simulink model "general_charger_2_precharge"  (R2013a)
settings: Solver=ode23  StartTime=0  StopTime=1.5  RelTol=1e-3
PreLoadFcn:
  | Ts =5e-6;
values from neighbouring files (symbols this model uses):
  ac_volt = 169    [charger_init.m]    (also in charger_init_simpl.m)
  acdc_on_time = 0.2    [charger_init.m]    (also in charger_init_simpl.m = 0)
  Cdc = 2e-3    (= 0.002)    [charger_init.m]    (also in charger_init_simpl.m)
  dcAd = dcinvexp*(eye(dcnstates) + (Ts/2)*dcAc)    [charger_init.m]    (also in charger_init_simpl.m)
  dcBd = dcinvexp*dcBc    [charger_init.m]    (also in charger_init_simpl.m)
  dcCd = dcCc*dcinvexp*Ts    [charger_init.m]    (also in charger_init_simpl.m)
  dcDd = dcCc*dcinvexp*dcBc*(Ts/2) + dcDc    [charger_init.m]    (also in charger_init_simpl.m)
  ESRCd = 70e-3    (= 0.07)    [charger_init.m]    (also in charger_init_simpl.m)
  ESRLdcdc = 0.1    [charger_init.m]    (also in charger_init_simpl.m)
  ESRLin = 0.2    [charger_init.m]    (also in charger_init_simpl.m = 0.1)
  Ldcdc = 1.3e-3    (= 0.0013)    [charger_init.m]    (also in charger_init_simpl.m = 0.0014)
  Lin = 1.5e-3    (= 0.0015)    [charger_init.m]    (also in charger_init_simpl.m = 0.001)
  P = 1.92e3    (= 1920)    [charger_init.m]    (also in charger_init_simpl.m)
  pre_charge_off = 0.2    [charger_init.m]
  pre_charge_r = 10    [charger_init.m]    (also in charger_init_simpl.m = 6)
  pre_charge_ramp = (dc_volt - Vdcmin)/(acdc_ramp_end_time - acdc_on_time)    (= 336.666666667)    [charger_init.m]    (also in charger_init_simpl.m = (dc_volt - Vdcmin)/(acdc_ramp_end_time - acdc_on_time))
  Q = 0    [charger_init.m]    (also in charger_init_simpl.m)
  Rbatt = 0.20    (= 0.2)    [charger_init.m]    (also in charger_init_simpl.m = 0.1)
  switch_Ts = 5e-5    (= 5e-05)    [charger_init.m]    (also in charger_init_simpl.m)
  sys_Ts = 5e-6    (= 5e-06)    [charger_init.m]    (also in charger_init_simpl.m)
  Vdcmin = ac_volt + 10    (= 179)    [charger_init.m]    (also in charger_init_simpl.m)
  voc = 105    [charger_init.m]    (also in charger_init_simpl.m)
undefined symbols (not defined in the file or in its folder): cpi
undefined symbols (not defined in the file): active_power_on, Ad, Bd, Cd, dc_volt, dcdc_cc_ref, dcdc_cv_ref, dcdc_iki, dcdc_ikp, dcdc_on, dcdc_vki, dcdc_vkp, Dd, dq_id_ki, dq_id_kp, dq_iq_ki, dq_iq_kp, dq_vdc_ki, dq_vdc_kp, dqQ_ki, dqQ_kp, P_ki, P_kp, pi_iac_ki, pi_iac_kp, pi_vdc_ki, pi_vdc_kp, piQ_ki, piQ_kp, pr_iac_kp, pr_pr_ki, pr_pr_kp, pr_vdc_ki, pr_vdc_kp, reactive_power_on
libraries: simulink_extras x165, powerlib x64, simulink x35, powerlib_meascontrol x11
(part 1 of 7)
settings Model: Creator=Administrator  LastModifiedBy=jfmorris
settings DataIOCC: SaveFinalState=on  SignalLoggingSaveFormat=ModelDataLogs
settings OptimizationCC: ExpressionDepthLimit=2147483647
settings DebuggingCC: FcnCallInpInsideContextMsg=UseLocalSettings  UnconnectedLineMsg=none
settings GRTTargetCC: CombineOutputUpdateFcns=off  GRTInterface=on

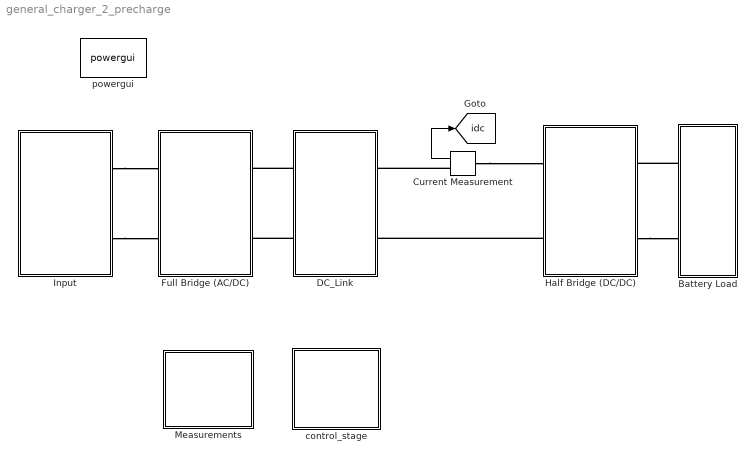
== system general_charger_2_precharge ==
  Battery Load : Subsystem
  Current Measurement : powerlib/Measurements/Current Measurement  PhasorSimulation=off  OutputType=Complex  PSBequivalent=0
  DC_Link : Subsystem
  Full Bridge (AC/DC) : Subsystem  mask{rsnub=50e3, csnub=0.33e-6, ron=1e-3, c_bridge=1e-6}
      mask prompts: rsnub "Snubber Resistance, ohms"; csnub "Snubber Capacitance, F"; ron "On Resistance, ohms"; c_bridge "Bridge Capacitance, F"
  Half Bridge (DC/DC) : Subsystem  mask{rsnub=50e3, csnub=1e-6, ron=1e-3, c_bridge=1e-6}
      mask prompts: rsnub "Snubber Resistance, ohms"; csnub "Snubber Capacitance, F"; ron "On Resistance, ohms"; c_bridge "Bridge Capacitance"
  Input : Subsystem
  Measurements : Subsystem
  control_stage : Subsystem
  powergui : powerlib/powergui  Priority=1  SimulationMode=Discrete  SolverType=Tustin  SampleTime=sys_Ts  frequency=60  SPID=off  DisableSnubberDevices=off  DisableRonSwitches=off  DisableVfSwitches=off  SwTol=0  Interpol=off  DisplayEquations=off  frequencyindice=0  Pbase=100e6  ErrMax=1e-4  Iterations=50  UnitsV=kV  UnitsW=MW  FunctionMessages=off  echomessages=off  HookPort=off  EnableUseOfTLC=off  x0status=blocks  RestoreLinks=warning  ResistiveCurrentMeasurement=off  Frange=[0:2:500]  Ylog=off  Xlog=on  ShowGrid=off  save=off  variable=ZData  ZoomFFT=off  StartTime=0.0  cycles=1  DisplayStyle=1  fundamental=60  FreqAxis=off  MaxFrequency=1000  frequencyindicesteady=1  RmsSteady=1  display=off  Ts=0  methode=off
  tag scope: idc=global
  wires:
  Current Measurement/1 -> [idc]
  connections:
  DC_Link/LConn1 -- Full Bridge (AC/DC)/RConn1
  DC_Link/LConn2 -- Full Bridge (AC/DC)/RConn2
  Battery Load/LConn1 -- Half Bridge (DC/DC)/LConn1
  Half Bridge (DC/DC)/LConn2 -- Battery Load/LConn2
  Input/RConn1 -- Full Bridge (AC/DC)/LConn1
  Input/RConn2 -- Full Bridge (AC/DC)/LConn2
  Current Measurement/RConn1 -- DC_Link/RConn1
  Current Measurement/LConn1 -- Half Bridge (DC/DC)/RConn1
  Half Bridge (DC/DC)/RConn2 -- DC_Link/RConn2

== system general_charger_2_precharge/Battery Load ==
  Battery (simple) : Subsystem  mask{batt_voc=50, rseries=0.25}
      mask prompts: batt_voc "open circuit voltage, V"; rseries "series resistance, ohms"
  Battery Model : Subsystem  mask{SOC=0.8, batt_voc=24, sorf=off}
      mask prompts: SOC "Current SOC, 0 for empty, 1 for full"; batt_voc "Open Circuit Voltage"; sorf "Quick Response? (check this box to simulate the battery charging and discharging in minutes instead of hours)"
  C : powerlib/Elements/Series RLC Branch  LConnTagsString=__new0  RConnTagsString=__new0  BranchType=C  Resistance=1  Inductance=1e-3  SetiL0=off  InitialCurrent=0  Capacitance=1e-3  Setx0=off  InitialVoltage=25  Measurements=None
  Current Measurement : powerlib/Measurements/Current Measurement  PhasorSimulation=off  OutputType=Complex  PSBequivalent=0
  DC Voltage Source : powerlib/Electrical Sources/DC Voltage Source  Amplitude=voc  Measurements=None
  ESR_C : powerlib/Elements/Series RLC Branch  LConnTagsString=__new0  RConnTagsString=__new0  BranchType=R  Resistance=30e-3  Inductance=1e-3  SetiL0=off  InitialCurrent=0  Capacitance=2.3e-3  Setx0=off  InitialVoltage=0  Measurements=None
  ESR_C1 : powerlib/Elements/Series RLC Branch  LConnTagsString=__new0  RConnTagsString=__new0  BranchType=R  Resistance=ESRLdcdc  Inductance=1e-3  SetiL0=off  InitialCurrent=0  Capacitance=2.3e-3  Setx0=off  InitialVoltage=0  Measurements=None
  L : powerlib/Elements/Series RLC Branch  LConnTagsString=__new0  RConnTagsString=__new0  BranchType=L  Resistance=1  Inductance=Ldcdc  SetiL0=off  InitialCurrent=0  Capacitance=1e-6  Setx0=off  InitialVoltage=0  Measurements=None
  Load : powerlib/Elements/Series RLC Branch  LConnTagsString=__new0  RConnTagsString=__new0  BranchType=R  Resistance=Rbatt  Inductance=1e-3  SetiL0=off  InitialCurrent=0  Capacitance=2.3e-3  Setx0=off  InitialVoltage=0  Measurements=None
  Voltage Measurement : powerlib/Measurements/Voltage Measurement  PhasorSimulation=off  OutputType=Complex  PSBequivalent=0
  V_batt+ : PMIOPort  Port=1  Side=Left
  V_batt- : PMIOPort  Port=2  Side=Left
  tag scope: idc_batt=global, vdc_batt=global
  wires:
  Voltage Measurement/1 -> [vdc_batt]
  Current Measurement/1 -> [idc_batt]
  connections:
  Voltage Measurement/LConn2 -- DC Voltage Source/LConn1 -- C/RConn1 -- V_batt-/RConn1
  L/LConn1 -- V_batt+/RConn1
  ESR_C/RConn1 -- C/LConn1
  Load/LConn1 -- Current Measurement/RConn1
  DC Voltage Source/RConn1 -- Load/RConn1
  Voltage Measurement/LConn1 -- Current Measurement/LConn1 -- ESR_C/LConn1 -- ESR_C1/RConn1
  L/RConn1 -- ESR_C1/LConn1

== system general_charger_2_precharge/DC_Link ==
  C : powerlib/Elements/Series RLC Branch  LConnTagsString=__new0  RConnTagsString=__new0  BranchType=C  Resistance=1  Inductance=1e-3  SetiL0=off  InitialCurrent=0  Capacitance=Cdc  Setx0=off  InitialVoltage=0  Measurements=None
  Current Measurement2 : powerlib/Measurements/Current Measurement  PhasorSimulation=off  OutputType=Complex  PSBequivalent=0
  ESR_C : powerlib/Elements/Series RLC Branch  LConnTagsString=__new0  RConnTagsString=__new0  BranchType=R  Resistance=ESRCd  Inductance=1e-3  SetiL0=off  InitialCurrent=0  Capacitance=2.3e-3  Setx0=off  InitialVoltage=0  Measurements=None
  ESR_C1 : powerlib/Elements/Series RLC Branch  LConnTagsString=__new0  RConnTagsString=__new0  BranchType=R  Resistance=pre_charge_r  Inductance=1e-3  SetiL0=off  InitialCurrent=0  Capacitance=2.3e-3  Setx0=off  InitialVoltage=0  Measurements=None
  IGBT/Diode3 : powerlib/Power Electronics/IGBT//Diode  Ron=1e-3  Rs=inf  Cs=0  Measurements=off
  Ideal Switch : powerlib/Power Electronics/Ideal Switch  Ron=0.001  Lon=0  IC=0  Rs=1e5  Cs=inf  Measurements=off
  Scope : Scope
      settings: SaveName=ScopeData9
  Step : Step  Time=pre_charge_off  SampleTime=0
  Voltage Measurement : powerlib/Measurements/Voltage Measurement  PhasorSimulation=off  OutputType=Complex  PSBequivalent=0
  Voltage Measurement1 : powerlib/Measurements/Voltage Measurement  PhasorSimulation=off  OutputType=Complex  PSBequivalent=0
  DC+In : PMIOPort  Port=1  Side=Left
  DC-In : PMIOPort  Port=2  Side=Left
  DC+Out : PMIOPort  Port=3  Side=Right
  DC-Out : PMIOPort  Port=4  Side=Right
  tag scope: i_cap=global, vdc_ideal=global
  wires:
  Current Measurement2/1 -> [i_cap]
  Voltage Measurement/1 -> [vdc_ideal]
  Voltage Measurement1/1 -> Scope/1
  Step/1 -> IGBT/Diode3/1
  connections:
  ESR_C/RConn1 -- C/LConn1
  C/RConn1 -- DC-Out/RConn1 -- Voltage Measurement/LConn2 -- DC-In/RConn1
  DC+Out/RConn1 -- Current Measurement2/LConn1 -- DC+In/RConn1
  ESR_C1/RConn1 -- Current Measurement2/RConn1 -- IGBT/Diode3/LConn1 -- Voltage Measurement1/LConn1
  Voltage Measurement/LConn1 -- IGBT/Diode3/RConn1 -- Voltage Measurement1/LConn2 -- ESR_C1/LConn1 -- ESR_C/LConn1

== system general_charger_2_precharge/Full Bridge (AC//DC) ==
  IGBT/Diode{,1..3} (4 alike) : powerlib/Power Electronics/IGBT//Diode  Ron=ron  Rs=inf  Cs=0  Measurements=off
  RC{,1..3} (4 alike) : powerlib/Elements/Parallel RLC Branch  LConnTagsString=a  RConnTagsString=__new0  BranchType=C  Resistance=100  Inductance=1e-3  SetiL0=off  InitialCurrent=0  Capacitance=csnub  Setx0=off  InitialVoltage=0  Measurements=None
  RC{8..11} (4 alike) : powerlib/Elements/Parallel RLC Branch  LConnTagsString=a  RConnTagsString=__new0  BranchType=C  Resistance=100  Inductance=1e-3  SetiL0=off  InitialCurrent=0  Capacitance=c_bridge  Setx0=off  InitialVoltage=0  Measurements=None
  RC{4..7} (4 alike) : powerlib/Elements/Parallel RLC Branch  LConnTagsString=a  RConnTagsString=__new0  BranchType=R  Resistance=rsnub  Inductance=1e-3  SetiL0=off  InitialCurrent=0  Capacitance=0.1e-6  Setx0=off  InitialVoltage=0  Measurements=None
  AC+ : PMIOPort  Port=1  Side=Left
  AC- : PMIOPort  Port=2  Side=Left
  DC+ : PMIOPort  Port=3  Side=Right
  DC- : PMIOPort  Port=4  Side=Right
  wires:
  [A] -> IGBT/Diode/1
  [B] -> IGBT/Diode1/1
  [C] -> IGBT/Diode3/1
  [D] -> IGBT/Diode2/1
  connections:
  IGBT/Diode/LConn1 -- RC10/LConn1 -- RC9/LConn1 -- RC7/LConn1 -- RC11/LConn1 -- RC8/LConn1 -- IGBT/Diode3/LConn1 -- RC5/LConn1 -- DC+/RConn1
  RC1/RConn1 -- AC+/RConn1 -- RC6/LConn1 -- IGBT/Diode1/LConn1 -- IGBT/Diode/RConn1
  IGBT/Diode2/RConn1 -- RC11/RConn1 -- RC8/RConn1 -- DC-/RConn1 -- RC10/RConn1 -- RC9/RConn1 -- IGBT/Diode1/RConn1 -- RC/RConn1 -- RC3/RConn1
  AC-/RConn1 -- IGBT/Diode3/RConn1 -- RC2/RConn1 -- RC4/LConn1 -- IGBT/Diode2/LConn1
  RC7/RConn1 -- RC1/LConn1
  RC6/RConn1 -- RC/LConn1
  RC4/RConn1 -- RC3/LConn1
  RC5/RConn1 -- RC2/LConn1

== system general_charger_2_precharge/Half Bridge (DC//DC) ==
  IGBT/Diode : powerlib/Power Electronics/IGBT//Diode  Ron=ron  Rs=inf  Cs=0  Measurements=off
  IGBT/Diode1 : powerlib/Power Electronics/IGBT//Diode  Ron=ron  Rs=inf  Cs=0  Measurements=off
  RC : powerlib/Elements/Parallel RLC Branch  LConnTagsString=a  RConnTagsString=__new0  BranchType=C  Resistance=100  Inductance=1e-3  SetiL0=off  InitialCurrent=0  Capacitance=csnub  Setx0=off  InitialVoltage=0  Measurements=None
  RC1 : powerlib/Elements/Parallel RLC Branch  LConnTagsString=a  RConnTagsString=__new0  BranchType=C  Resistance=100  Inductance=1e-3  SetiL0=off  InitialCurrent=0  Capacitance=csnub  Setx0=off  InitialVoltage=0  Measurements=None
  RC2 : powerlib/Elements/Parallel RLC Branch  LConnTagsString=a  RConnTagsString=__new0  BranchType=C  Resistance=100  Inductance=1e-3  SetiL0=off  InitialCurrent=0  Capacitance=c_bridge  Setx0=off  InitialVoltage=0  Measurements=None
  RC3 : powerlib/Elements/Parallel RLC Branch  LConnTagsString=a  RConnTagsString=__new0  BranchType=C  Resistance=100  Inductance=1e-3  SetiL0=off  InitialCurrent=0  Capacitance=c_bridge  Setx0=off  InitialVoltage=0  Measurements=None
  Snubber2 : powerlib/Elements/Series RLC Branch  LConnTagsString=__new0  RConnTagsString=__new0  BranchType=R  Resistance=rsnub  Inductance=1e-3  SetiL0=off  InitialCurrent=0  Capacitance=0.1e-6  Setx0=off  InitialVoltage=0  Measurements=None
  Snubber3 : powerlib/Elements/Series RLC Branch  LConnTagsString=__new0  RConnTagsString=__new0  BranchType=R  Resistance=rsnub  Inductance=1e-3  SetiL0=off  InitialCurrent=0  Capacitance=0.1e-6  Setx0=off  InitialVoltage=0  Measurements=None
  DC_batt+ : PMIOPort  Port=1  Side=Left
  DC_batt- : PMIOPort  Port=2  Side=Left
  DC_link+ : PMIOPort  Port=3  Side=Right
  DC_link- : PMIOPort  Port=4  Side=Right
  wires:
  [E] -> IGBT/Diode/1
  [F] -> IGBT/Diode1/1
  connections:
  IGBT/Diode/LConn1 -- RC3/LConn1 -- RC2/LConn1 -- DC_link+/RConn1 -- Snubber3/LConn1
  RC1/RConn1 -- DC_batt+/RConn1 -- Snubber2/LConn1 -- IGBT/Diode1/LConn1 -- IGBT/Diode/RConn1
  DC_link-/RConn1 -- DC_batt-/RConn1 -- RC3/RConn1 -- RC2/RConn1 -- IGBT/Diode1/RConn1 -- RC/RConn1
  Snubber3/RConn1 -- RC1/LConn1
  Snubber2/RConn1 -- RC/LConn1

== system general_charger_2_precharge/Input ==
  C2 : powerlib/Elements/Series RLC Branch  LConnTagsString=__new0  RConnTagsString=__new0  BranchType=R  Resistance=1e-3  Inductance=1e-3  SetiL0=off  InitialCurrent=0  Capacitance=cpi  Setx0=off  InitialVoltage=0  Measurements=None
  Current Measurement : powerlib/Measurements/Current Measurement  PhasorSimulation=off  OutputType=Complex  PSBequivalent=0
  ESR_L : powerlib/Elements/Series RLC Branch  LConnTagsString=__new0  RConnTagsString=__new0  BranchType=R  Resistance=ESRLin  Inductance=1e-3  SetiL0=off  InitialCurrent=0  Capacitance=1e-6  Setx0=off  InitialVoltage=0  Measurements=None
  L : powerlib/Elements/Series RLC Branch  LConnTagsString=__new0  RConnTagsString=__new0  BranchType=L  Resistance=1  Inductance=Lin  SetiL0=off  InitialCurrent=0  Capacitance=1e-6  Setx0=off  InitialVoltage=0  Measurements=None
  Power Line Filter : Subsystem  mask{cx=1e-6, rx=330e3, lchoke=2e-3}
      mask prompts: cx "X Capacitance, F"; rx "X Resistance, ohms"; lchoke "Choke Inductance, H"
  RsenseVac : powerlib/Elements/Series RLC Branch  LConnTagsString=__new0  RConnTagsString=__new0  BranchType=R  Resistance=10000  Inductance=1e-3  SetiL0=off  InitialCurrent=0  Capacitance=1e-6  Setx0=off  InitialVoltage=0  Measurements=None
  Voltage Measurement1 : powerlib/Measurements/Voltage Measurement  PhasorSimulation=off  OutputType=Complex  PSBequivalent=0
  Voltage Measurement3 : powerlib/Measurements/Voltage Measurement  PhasorSimulation=off  OutputType=Complex  PSBequivalent=0
  Vs : powerlib/Electrical Sources/AC Voltage Source  Amplitude=ac_volt  Phase=0  Frequency=60  SampleTime=0  Measurements=None
  Out+ : PMIOPort  Port=1  Side=Right
  Out- : PMIOPort  Port=2  Side=Right
  tag scope: Is=global, Vc=global, vs_ideal=global
  wires:
  Current Measurement/1 -> [Is]
  Voltage Measurement3/1 -> [Vc]
  Voltage Measurement1/1 -> [vs_ideal]
  connections:
  RsenseVac/LConn1 -- Power Line Filter/RConn1 -- L/LConn1
  Out-/RConn1 -- Power Line Filter/RConn2 -- RsenseVac/RConn1 -- Voltage Measurement3/LConn2
  Out+/RConn1 -- Voltage Measurement3/LConn1 -- Current Measurement/RConn1
  ESR_L/RConn1 -- Current Measurement/LConn1
  ESR_L/LConn1 -- L/RConn1
  Voltage Measurement1/LConn2 -- Power Line Filter/LConn2 -- Vs/LConn1
  Voltage Measurement1/LConn1 -- Vs/RConn1 -- C2/LConn1
  C2/RConn1 -- Power Line Filter/LConn1

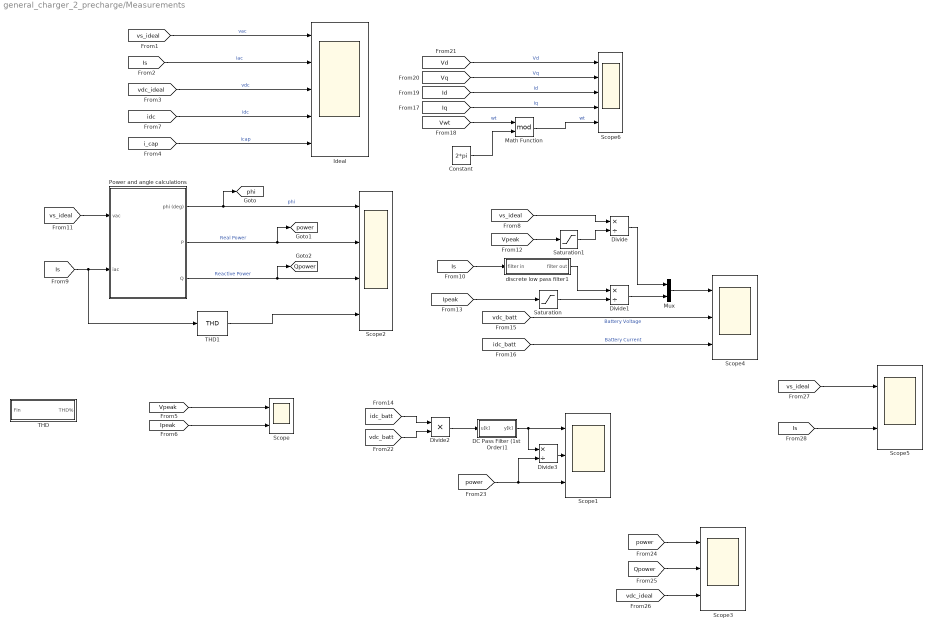
== system general_charger_2_precharge/Measurements ==
  Constant : Constant  Value=2*pi
  DC Pass Filter (1st Order)1 : Subsystem  mask{dc_filter_Ts=5e-5}
      mask prompts: dc_filter_Ts "Sample Time"
      mask help: Low Pass Filter to provide unity gain and 0 phase shift at DC
  Divide : Product  Inputs=*/
  Divide1 : Product  Inputs=*/
  Divide2 : Product  Inputs=**
  Divide3 : Product  Inputs=*/
  Ideal : Scope  NumInputPorts=5
      settings: TimeRange=0.5  YMin=-175~-15~373~-4~-5  YMax=175~15~389~2~6  SaveName=ScopeData8
  Math Function : Math  Operator=mod  SaturateOnIntegerOverflow=on
  Mux : Mux  Inputs=2
  Power and angle calculations : Subsystem
  Saturation : Saturate  UpperLimit=inf  LowerLimit=1
  Saturation1 : Saturate  UpperLimit=inf  LowerLimit=1
  Scope : Scope  NumInputPorts=2
      settings: YMin=-70~-70  YMax=30~40  SaveName=ScopeData6
  Scope1 : Scope  NumInputPorts=3
      settings: ShowLegends=on  TimeRange=0.3  YMin=-6.5~0~-125  YMax=1~1~325  SaveName=is_vs_  MaxDataPoints=50000
  Scope2 : Scope  NumInputPorts=4
      settings: ShowLegends=on  TimeRange=0.5  YMin=-43.4~3350~-3180~0.0525  YMax=-42.1~3430~-3095~0.058  SaveName=is_vs_2  MaxDataPoints=50000
  Scope3 : Scope  NumInputPorts=3
      settings: ShowLegends=on  TimeRange=0.3  YMin=4047.5~-6.5~367  YMax=4087.5~-0.5~388  SaveName=power_vdc_1  MaxDataPoints=50000
  Scope4 : Scope  NumInputPorts=3
      settings: ShowLegends=on  TimeRange=0.3  YMin=-0.9~76.225~42.25  YMax=0.5~76.5~45  SaveName=i_v_batt_1  MaxDataPoints=50000
  Scope5 : Scope  NumInputPorts=2
      settings: ShowLegends=on  TimeRange=0.3  YMin=-0.9~76.225  YMax=0.5~76.5  SaveName=i_v_ac_1  MaxDataPoints=50000
  Scope6 : Scope  NumInputPorts=5
      settings: ShowLegends=on  YMin=169.05~-0.05~18~-7.5~316  YMax=169.12~0.06~30~7.5~324  SaveName=ScopeData3
  THD : Subsystem  mask{calc_type=THD, S=3.3e3, vrms=120}
      mask prompts: calc_type "calculation type"; S "controller kva rating"; vrms "rms grid voltage"
      mask TypeOptions calc_type: TDD | THD
  THD1 : powerlib_meascontrol/Measurements/THD  Freq=60  Ts=switch_Ts
  discrete low pass filter1 : Subsystem
      mask Display: disp('fitler');
  tag scope: Qpower=global, phi=global, power=global
  wires:
  [Vq] -> Scope6/2  "Vq"
  [Iq] -> Scope6/4  "Iq"
  [Id] -> Scope6/3  "Id"
  [Vd] -> Scope6/1  "Vd"
  [vs_ideal] -> Power and angle calculations/1(vac)
  Power and angle calculations/1(phi (deg)) -> [phi], Scope2/1  "phi"
  Power and angle calculations/2(P) -> [power], Scope2/2  "Real Power"
  Power and angle calculations/3(Q) -> Scope2/3, [Qpower]  "Reactive Power"
  [vs_ideal] -> Ideal/1  "vac"
  [Is] -> Ideal/2  "iac"
  [vdc_ideal] -> Ideal/3  "vdc"
  [Is] -> THD1/1, Power and angle calculations/2(iac)
  [idc] -> Ideal/4  "idc"
  [vdc_batt] -> Scope4/2  "Battery Voltage"
  [idc_batt] -> Scope4/3  "Battery Current"
  [vs_ideal] -> Divide/1
  [Vpeak] -> Saturation1/1
  [Ipeak] -> Saturation/1
  Divide/1 -> Mux/1
  Divide1/1 -> Mux/2
  [Vwt] -> Math Function/1  "wt"
  Constant/1 -> Math Function/2
  Math Function/1 -> Scope6/5  "wt"
  Mux/1 -> Scope4/1
  [Is] -> discrete low pass filter1/1(filter in)
  discrete low pass filter1/1(filter out) -> Divide1/1
  [i_cap] -> Ideal/5  "icap"
  [Ipeak] -> Scope/2
  [Vpeak] -> Scope/1
  Saturation/1 -> Divide1/2
  Saturation1/1 -> Divide/2
  THD1/1 -> Scope2/4
  [idc_batt] -> Divide2/1
  [vdc_batt] -> Divide2/2
  Divide2/1 -> DC Pass Filter (1st Order)1/1(u[k])
  DC Pass Filter (1st Order)1/1(y[k]) -> Divide3/1, Scope1/1
  Divide3/1 -> Scope1/2
  [power] -> Divide3/2, Scope1/3
  [power] -> Scope3/1
  [Qpower] -> Scope3/2
  [vdc_ideal] -> Scope3/3
  [Is] -> Scope5/2
  [vs_ideal] -> Scope5/1

== system general_charger_2_precharge/control_stage ==
  AC/DC Control : Subsystem  mask{acdc_control=dq}
      mask prompts: acdc_control "ac/dc controller"
      mask TypeOptions acdc_control: pi | dq | pr
  DC/DC Control : Subsystem  mask{mode=Constant Power, cc_ref=dcdc_cc_ref, cv_ref=dcdc_cv_ref, cc_kp=dcdc_iki, cc_ki=dcdc_ikp, vc_ki=dcdc_vki, vc_kp=dcdc_vkp, turn_on=dcdc_on, pturn_on=active_power_on, Ts=switch_Ts}
      mask prompts: mode "battery operation mode"; cc_ref "CC reference (A)"; cv_ref "CV reference (V)"; cc_kp "current controller integral gain"; cc_ki "current controller proportional gain"; vc_ki "voltage controller integral gain"; vc_kp "voltage controller proportional gain"; turn_on "DC/DC Turn On time (s)"; pturn_on "Active Power Control Turn on time (s)"; Ts "Sample Time"
      mask TypeOptions mode: Constant Voltage | Constant Current | Constant Power
  wires:
  [idc_batt] -> DC/DC Control/1(Ibatt)
  [vdc_batt] -> DC/DC Control/2(Vbatt)
  [vdc_ideal] -> AC/DC Control/2(vdc)
  [vs_ideal] -> AC/DC Control/1(vac)
  [Is] -> AC/DC Control/3(iac)

== system general_charger_2_precharge/Battery Load/Battery (simple) ==
  ESR_C2 : powerlib/Elements/Series RLC Branch  LConnTagsString=__new0  RConnTagsString=__new0  BranchType=R  Resistance=rseries  Inductance=1e-3  SetiL0=off  InitialCurrent=0  Capacitance=2.3e-3  Setx0=off  InitialVoltage=0  Measurements=None
  voc : powerlib/Electrical Sources/DC Voltage Source  Amplitude=batt_voc  Measurements=None
  + : PMIOPort  Port=1  Side=Left
  - : PMIOPort  Port=2  Side=Left
  connections:
  ESR_C2/LConn1 -- voc/RConn1
  ESR_C2/RConn1 -- +/RConn1
  voc/LConn1 -- -/RConn1

== system general_charger_2_precharge/Battery Load/Battery Model ==
  c_transient_long : powerlib/Elements/Series RLC Branch  LConnTagsString=__new0  RConnTagsString=__new0  BranchType=C  Resistance=0.01  Inductance=1e-3  SetiL0=off  InitialCurrent=0  Capacitance=-6056*exp(-27.12*SOC)*(1-sorf) + 4475 - 4474*sorf  Setx0=off  InitialVoltage=0  Measurements=None
  c_transient_short : powerlib/Elements/Series RLC Branch  LConnTagsString=__new0  RConnTagsString=__new0  BranchType=C  Resistance=0.01  Inductance=1e-3  SetiL0=off  InitialCurrent=0  Capacitance=-752.9*exp(-13.51*SOC)*(1-sorf) + 703.6 + 703*sorf  Setx0=off  InitialVoltage=0  Measurements=None
  r_series : powerlib/Elements/Series RLC Branch  LConnTagsString=__new0  RConnTagsString=__new0  BranchType=R  Resistance=0.1563*exp(-24.37*SOC*(1-sorf))+0.07446  Inductance=1e-3  SetiL0=off  InitialCurrent=0  Capacitance=2.3e-3  Setx0=off  InitialVoltage=0  Measurements=None
  r_transient_long : powerlib/Elements/Series RLC Branch  LConnTagsString=__new0  RConnTagsString=__new0  BranchType=R  Resistance=6.603*exp(-155.2*SOC*(1-sorf)) + 0.04984  Inductance=1e-3  SetiL0=off  InitialCurrent=0  Capacitance=2.3e-3  Setx0=off  InitialVoltage=0  Measurements=None
  r_transient_short : powerlib/Elements/Series RLC Branch  LConnTagsString=__new0  RConnTagsString=__new0  BranchType=R  Resistance=0.3208*exp(-29.14*SOC*(1-sorf)) + 0.04669  Inductance=1e-3  SetiL0=off  InitialCurrent=0  Capacitance=2.3e-3  Setx0=off  InitialVoltage=0  Measurements=None
  voc : powerlib/Electrical Sources/DC Voltage Source  Amplitude=batt_voc  Measurements=None
  + : PMIOPort  Port=1  Side=Left
  - : PMIOPort  Port=2  Side=Left
  connections:
  r_transient_short/RConn1 -- c_transient_short/RConn1 -- +/RConn1
  voc/LConn1 -- -/RConn1
  r_transient_long/RConn1 -- c_transient_long/RConn1 -- c_transient_short/LConn1 -- r_transient_short/LConn1
  r_transient_long/LConn1 -- r_series/RConn1 -- c_transient_long/LConn1
  r_series/LConn1 -- voc/RConn1

== system general_charger_2_precharge/Input/Power Line Filter ==
  C : powerlib/Elements/Series RLC Branch  LConnTagsString=__new0  RConnTagsString=__new0  BranchType=C  Resistance=1  Inductance=1e-3  SetiL0=off  InitialCurrent=0  Capacitance=cx  Setx0=off  InitialVoltage=0  Measurements=None
  C1 : powerlib/Elements/Series RLC Branch  LConnTagsString=__new0  RConnTagsString=__new0  BranchType=C  Resistance=1  Inductance=1e-3  SetiL0=off  InitialCurrent=0  Capacitance=cx  Setx0=off  InitialVoltage=0  Measurements=None
  C2 : powerlib/Elements/Series RLC Branch  LConnTagsString=__new0  RConnTagsString=__new0  BranchType=R  Resistance=rx  Inductance=1e-3  SetiL0=off  InitialCurrent=0  Capacitance=cpi  Setx0=off  InitialVoltage=0  Measurements=None
  Choke : powerlib/Elements/Mutual Inductance  LConnTagsString=a|b  RConnTagsString=A|B  TypeOfMutual=Two or three windings with equal mutual terms  NumberOfWindings=2  SelfImpedance1=[0 lchoke]  SelfImpedance2=[0 lchoke]  ThreeWindings=off  SelfImpedance3=[ 1.1 1.1e-03]  MutualImpedance=[0 lchoke*0.99999]  InductanceMatrix="[0 1e-6 ; 1e-6  0]"  ResistanceMatrix=[0 0; 0 0]  Measurements=None
      settings: AttributesFormatString=\n
  Voltage Measurement3 : powerlib/Measurements/Voltage Measurement  PhasorSimulation=off  OutputType=Complex  PSBequivalent=0
  Voltage Measurement4 : powerlib/Measurements/Voltage Measurement  PhasorSimulation=off  OutputType=Complex  PSBequivalent=0
  PLF IN + : PMIOPort  Port=1  Side=Left
  PLF OUT + : PMIOPort  Port=2  Side=Right
  PLF IN - : PMIOPort  Port=3  Side=Left
  PLF OUT - : PMIOPort  Port=4  Side=Right
  tag scope: vchoke1=global, vchoke2=global
  wires:
  Voltage Measurement3/1 -> [vchoke1]
  Voltage Measurement4/1 -> [vchoke2]
  connections:
  PLF IN +/RConn1 -- C2/LConn1 -- Voltage Measurement3/LConn1 -- Choke/LConn1 -- C/LConn1
  PLF IN -/RConn1 -- C2/RConn1 -- Voltage Measurement4/LConn1 -- Choke/LConn2 -- C/RConn1
  Voltage Measurement3/LConn2 -- Choke/RConn1 -- C1/LConn1 -- PLF OUT +/RConn1
  Voltage Measurement4/LConn2 -- Choke/RConn2 -- C1/RConn1 -- PLF OUT -/RConn1

== system general_charger_2_precharge/Measurements/DC Pass Filter (1st Order)1 ==
  u[k] : Inport
  A : Gain  Gain=dcAd
  B : Gain  Gain=dcBd
  C : Gain  Gain=dcCd
  D : Gain  Gain=dcDd
  Delay : Delay  DelayLength=1  InitialCondition=0  SampleTime=5e-5
  Sum : Sum  Inputs=|++
  Sum1 : Sum  Inputs=|++
  y[k] : Outport
  wires:
  B/1 -> Sum/1
  u[k]/1 -> D/1, B/1
  Sum1/1 -> y[k]/1
  Delay/1 -> A/1, C/1
  Sum/1 -> Delay/1
  D/1 -> Sum1/1
  A/1 -> Sum/2
  C/1 -> Sum1/2

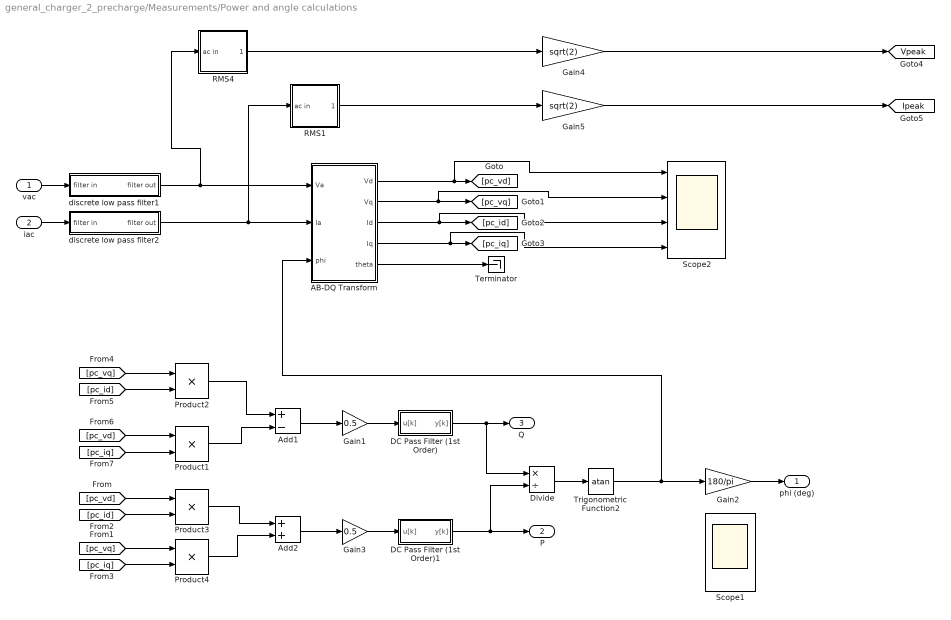
== system general_charger_2_precharge/Measurements/Power and angle calculations ==
  vac : Inport
  iac : Inport  Port=2
  AB-DQ Transform : Subsystem
  Add1 : Sum  Inputs=+-
  Add2 : Sum
  DC Pass Filter (1st Order) : Subsystem  mask{dc_filter_Ts=5e-5}
      mask prompts: dc_filter_Ts "Sample Time"
      mask help: Low Pass Filter to provide unity gain and 0 phase shift at DC
  DC Pass Filter (1st Order)1 : Subsystem  mask{dc_filter_Ts=5e-5}
      mask prompts: dc_filter_Ts "Sample Time"
      mask help: Low Pass Filter to provide unity gain and 0 phase shift at DC
  Divide : Product  Inputs=*/
  Gain1 : Gain  Gain=0.5
  Gain2 : Gain  Gain=180/pi
  Gain3 : Gain  Gain=0.5
  Gain4 : Gain  Gain=sqrt(2)
  Gain5 : Gain  Gain=sqrt(2)
  Product{1..4} (4 alike) : Product  RndMeth=Zero
  RMS1 : Subsystem  mask{f=60, rms_Ts=4e-4}
      mask prompts: f "Fundamental Frequency"; rms_Ts "Sample Time"
      mask init:
      | SpC=1/f/rms_Ts;
      | RSpC=ceil(SpC);
      | Delay=RSpC*rms_Ts;
      | Corr1=(SpC-RSpC)/2;
      | Corr2=(SpC-RSpC)/SpC;
      | K1=Corr1*Corr2;
      | K2=Corr2 + Corr1*Corr2;
      mask Display: disp('RMS')
  RMS4 : Subsystem  mask{f=60, rms_Ts=4e-4}
      mask prompts: f "Fundamental Frequency"; rms_Ts "Sample Time"
      mask init:
      | SpC=1/f/rms_Ts;
      | RSpC=ceil(SpC);
      | Delay=RSpC*rms_Ts;
      | Corr1=(SpC-RSpC)/2;
      | Corr2=(SpC-RSpC)/SpC;
      | K1=Corr1*Corr2;
      | K2=Corr2 + Corr1*Corr2;
      mask Display: disp('RMS')
  Scope1 : Scope
      settings: ShowLegends=on  YMin=2500  YMax=3000  SaveName=Power
  Scope2 : Scope  NumInputPorts=4
      settings: YMin=-5~-5~-5~-5  YMax=5~5~5~5  SaveName=ScopeData17
  Terminator : Terminator
  Trigonometric Function2 : Trigonometry  Operator=atan
  discrete low pass filter1 : Subsystem
      mask Display: disp('fitler');
  discrete low pass filter2 : Subsystem
      mask Display: disp('fitler');
  phi (deg) : Outport
  P : Outport  Port=2
  Q : Outport  Port=3
  tag scope: Ipeak=global, Vpeak=global
  wires:
  Product3/1 -> Add2/1
  Product2/1 -> Add1/1
  Divide/1 -> Trigonometric Function2/1
  Trigonometric Function2/1 -> AB-DQ Transform/3(phi), Gain2/1
  [pc_vd] -> Product1/1
  [pc_iq] -> Product1/2
  [pc_id] -> Product3/2
  [pc_vd] -> Product3/1
  [pc_vq] -> Product4/1
  [pc_iq] -> Product4/2
  [pc_vq] -> Product2/1
  [pc_id] -> Product2/2
  Gain2/1 -> phi (deg)/1
  vac/1 -> discrete low pass filter1/1(filter in)
  AB-DQ Transform/1(Vd) -> Scope2/1, [pc_vd]
  AB-DQ Transform/2(Vq) -> Scope2/2, [pc_vq]
  AB-DQ Transform/3(Id) -> Scope2/3, [pc_id]
  AB-DQ Transform/4(Iq) -> Scope2/4, [pc_iq]
  AB-DQ Transform/5(theta) -> Terminator/1
  Gain4/1 -> [Vpeak]
  Gain5/1 -> [Ipeak]
  Product1/1 -> Add1/2
  Product4/1 -> Add2/2
  RMS1/1(rms out) -> Gain5/1
  RMS4/1(rms out) -> Gain4/1
  iac/1 -> discrete low pass filter2/1(filter in)
  discrete low pass filter2/1(filter out) -> RMS1/1(ac in), AB-DQ Transform/2(Ia)
  discrete low pass filter1/1(filter out) -> RMS4/1(ac in), AB-DQ Transform/1(Va)
  DC Pass Filter (1st Order)1/1(y[k]) -> Divide/2, P/1
  DC Pass Filter (1st Order)/1(y[k]) -> Divide/1, Q/1
  Add2/1 -> Gain3/1
  Add1/1 -> Gain1/1
  Gain1/1 -> DC Pass Filter (1st Order)/1(u[k])
  Gain3/1 -> DC Pass Filter (1st Order)1/1(u[k])

== system general_charger_2_precharge/Measurements/THD ==
  Fin : Inport
  Add : Sum  Inputs=+-
  Constant : Constant  Value=S/vrms
  Constant1 : Constant  Value=calc_type
  Divide : Product  Inputs=*/
  Gain : Gain  Gain=100
  Product : Product
  Product1 : Product
  RMS1 : Subsystem  mask{f=60, rms_Ts=4e-4}
      mask prompts: f "Fundamental Frequency"; rms_Ts "Sample Time"
      mask init:
      | SpC=1/f/rms_Ts;
      | RSpC=ceil(SpC);
      | Delay=RSpC*rms_Ts;
      | Corr1=(SpC-RSpC)/2;
      | Corr2=(SpC-RSpC)/SpC;
      | K1=Corr1*Corr2;
      | K2=Corr2 + Corr1*Corr2;
      mask Display: disp('RMS')
  RMS4 : Subsystem  mask{f=60, rms_Ts=4e-4}
      mask prompts: f "Fundamental Frequency"; rms_Ts "Sample Time"
      mask init:
      | SpC=1/f/rms_Ts;
      | RSpC=ceil(SpC);
      | Delay=RSpC*rms_Ts;
      | Corr1=(SpC-RSpC)/2;
      | Corr2=(SpC-RSpC)/SpC;
      | K1=Corr1*Corr2;
      | K2=Corr2 + Corr1*Corr2;
      mask Display: disp('RMS')
  Saturation : Saturate  UpperLimit=inf  LowerLimit=0.1
  Saturation1 : Saturate  UpperLimit=inf  LowerLimit=0
  Scope : Scope  NumInputPorts=4
      settings: YMin=-5~-5~-5~-5  YMax=5~5~5~5  SaveName=ScopeData19
  Scope1 : Scope  NumInputPorts=4
      settings: YMin=-5~-5~-5~-5  YMax=5~5~5~5  SaveName=ScopeData20
  Sqrt : Sqrt  SaturateOnIntegerOverflow=on
  Switch : Switch  Threshold=1.5
  discrete low pass filter1 : Subsystem
  THD% : Outport
  wires:
  Product1/1 -> Scope/4, Add/2
  Sqrt/1 -> Scope1/3, Divide/1
  Add/1 -> Scope1/1, Saturation1/1
  Saturation1/1 -> Scope1/2, Sqrt/1
  Saturation/1 -> Divide/2
  Divide/1 -> Scope1/4, Gain/1
  RMS4/1(rms out) -> Scope/1, Product/2, Product/1  "F"
  RMS1/1(rms out) -> Scope/2, Switch/1, Product1/2, Product1/1  "F1"
  Fin/1 -> RMS4/1(ac in), discrete low pass filter1/1(filter in)
  discrete low pass filter1/1(filter out) -> RMS1/1(ac in)
  Gain/1 -> THD%/1
  Switch/1 -> Saturation/1
  Constant/1 -> Switch/3
  Constant1/1 -> Switch/2
  Product/1 -> Scope/3, Add/1

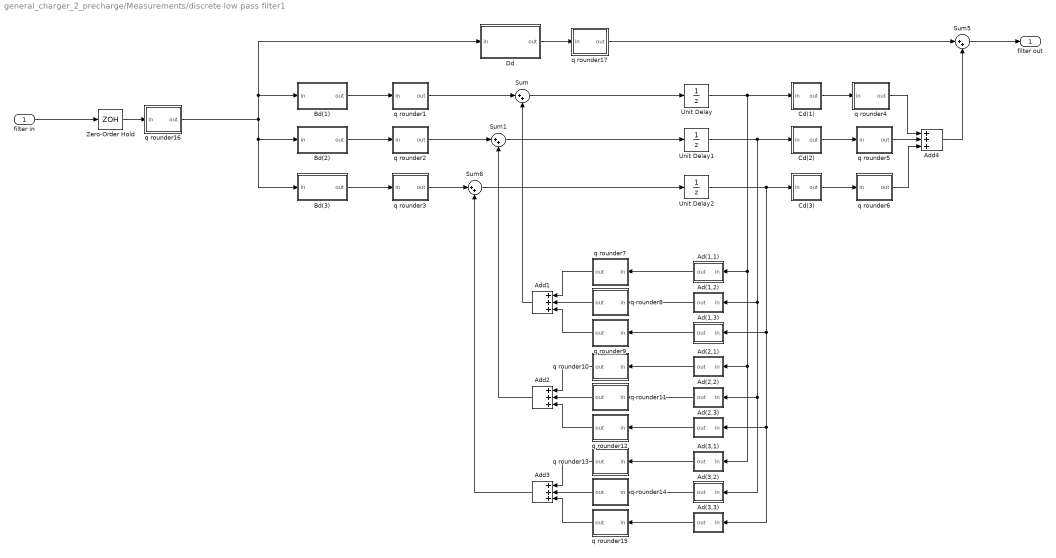
== system general_charger_2_precharge/Measurements/discrete low pass filter1 ==
  filter in : Inport
  Ad(1,1) : Subsystem  mask{variable=Ad(1,1), nQ=29, maxRange=4}
      mask prompts: variable "state-space variable"; nQ "q value"; maxRange "max range"
      mask Display: disp(nQ)
  Ad(1,2) : Subsystem  mask{variable=Ad(1,2), nQ=23, maxRange=256}
      mask prompts: variable "state-space variable"; nQ "q value"; maxRange "max range"
      mask Display: disp(nQ)
  Ad(1,3) : Subsystem  mask{variable=Ad(1,3), nQ=14, maxRange=131072}
      mask prompts: variable "state-space variable"; nQ "q value"; maxRange "max range"
      mask Display: disp(nQ)
  Ad(2,1) : Subsystem  mask{variable=Ad(2,1), nQ=30, maxRange=2}
      mask prompts: variable "state-space variable"; nQ "q value"; maxRange "max range"
      mask Display: disp(nQ)
  Ad(2,2) : Subsystem  mask{variable=Ad(2,2), nQ=29, maxRange=4}
      mask prompts: variable "state-space variable"; nQ "q value"; maxRange "max range"
      mask Display: disp(nQ)
  Ad(2,3) : Subsystem  mask{variable=Ad(2,3), nQ=29, maxRange=4}
      mask prompts: variable "state-space variable"; nQ "q value"; maxRange "max range"
      mask Display: disp(nQ)
  Ad(3,1) : Subsystem  mask{variable=Ad(3,1), nQ=30, maxRange=2}
      mask prompts: variable "state-space variable"; nQ "q value"; maxRange "max range"
      mask Display: disp(nQ)
  Ad(3,2) : Subsystem  mask{variable=Ad(3,2), nQ=30, maxRange=2}
      mask prompts: variable "state-space variable"; nQ "q value"; maxRange "max range"
      mask Display: disp(nQ)
  Ad(3,3) : Subsystem  mask{variable=Ad(3,3), nQ=29, maxRange=4}
      mask prompts: variable "state-space variable"; nQ "q value"; maxRange "max range"
      mask Display: disp(nQ)
  Add{1..4} (4 alike) : Sum  Inputs=+++
  Bd(1) : Subsystem  mask{variable=Bd(1), nQ=29, maxRange=4}
      mask prompts: variable "state-space variable"; nQ "q value"; maxRange "max range"
      mask Display: disp(nQ)
  Bd(2) : Subsystem  mask{variable=Bd(2), nQ=30, maxRange=2}
      mask prompts: variable "state-space variable"; nQ "q value"; maxRange "max range"
      mask Display: disp(nQ)
  Bd(3) : Subsystem  mask{variable=Bd(3), nQ=30, maxRange=2}
      mask prompts: variable "state-space variable"; nQ "q value"; maxRange "max range"
      mask Display: disp(nQ)
  Cd(1) : Subsystem  mask{variable=Cd(1), nQ=30, maxRange=2}
      mask prompts: variable "state-space variable"; nQ "q value"; maxRange "max range"
      mask Display: disp(nQ)
  Cd(2) : Subsystem  mask{variable=Cd(2), nQ=23, maxRange=256}
      mask prompts: variable "state-space variable"; nQ "q value"; maxRange "max range"
      mask Display: disp(nQ)
  Cd(3) : Subsystem  mask{variable=Cd(3), nQ=15, maxRange=65536}
      mask prompts: variable "state-space variable"; nQ "q value"; maxRange "max range"
      mask Display: disp(nQ)
  Dd : Subsystem  mask{variable=Dd, nQ=30, maxRange=2}
      mask prompts: variable "state-space variable"; nQ "q value"; maxRange "max range"
      mask Display: disp(nQ)
  Sum{,1,5..6} (4 alike) : Sum  Inputs=|++
  Unit Delay : UnitDelay  SampleTime=5e-5
  Unit Delay1 : UnitDelay  SampleTime=5e-5
  Unit Delay2 : UnitDelay  SampleTime=5e-5
  Zero-Order Hold : ZeroOrderHold  SampleTime=5e-5
  q rounder1 : Subsystem  mask{q=22, range=512}
      mask prompts: q "q value"; range "q range"
      mask Display: disp(q)
  q rounder10 : Subsystem  mask{q=30, range=2}
      mask prompts: q "q value"; range "q range"
      mask Display: disp(q)
  q rounder11 : Subsystem  mask{q=30, range=2}
      mask prompts: q "q value"; range "q range"
      mask Display: disp(q)
  q rounder12 : Subsystem  mask{q=30, range=2}
      mask prompts: q "q value"; range "q range"
      mask Display: disp(q)
  q rounder13 : Subsystem  mask{q=30, range=2}
      mask prompts: q "q value"; range "q range"
      mask Display: disp(q)
  q rounder14 : Subsystem  mask{q=30, range=2}
      mask prompts: q "q value"; range "q range"
      mask Display: disp(q)
  q rounder15 : Subsystem  mask{q=30, range=2}
      mask prompts: q "q value"; range "q range"
      mask Display: disp(q)
  q rounder16 : Subsystem  mask{q=19, range=4096}
      mask prompts: q "q value"; range "q range"
      mask Display: disp(q)
  q rounder17 : Subsystem  mask{q=30, range=2}
      mask prompts: q "q value"; range "q range"
      mask Display: disp(q)
  q rounder2 : Subsystem  mask{q=30, range=2}
      mask prompts: q "q value"; range "q range"
      mask Display: disp(q)
  q rounder3 : Subsystem  mask{q=30, range=2}
      mask prompts: q "q value"; range "q range"
      mask Display: disp(q)
  q rounder4 : Subsystem  mask{q=19, range=4096}
      mask prompts: q "q value"; range "q range"
      mask Display: disp(q)
  q rounder5 : Subsystem  mask{q=19, range=4096}
      mask prompts: q "q value"; range "q range"
      mask Display: disp(q)
  q rounder6 : Subsystem  mask{q=19, range=4096}
      mask prompts: q "q value"; range "q range"
      mask Display: disp(q)
  q rounder7 : Subsystem  mask{q=22, range=512}
      mask prompts: q "q value"; range "q range"
      mask Display: disp(q)
  q rounder8 : Subsystem  mask{q=22, range=512}
      mask prompts: q "q value"; range "q range"
      mask Display: disp(q)
  q rounder9 : Subsystem  mask{q=22, range=512}
      mask prompts: q "q value"; range "q range"
      mask Display: disp(q)
  filter out : Outport
  wires:
  Sum/1 -> Unit Delay/1
  Sum1/1 -> Unit Delay1/1
  Unit Delay/1 -> Ad(3,1)/1(in), Ad(2,1)/1(in), Ad(1,1)/1(in), Cd(1)/1(in)
  Unit Delay1/1 -> Ad(3,2)/1(in), Ad(2,2)/1(in), Ad(1,2)/1(in), Cd(2)/1(in)
  Dd/1(out) -> q rounder17/1(in)
  Sum5/1 -> filter out/1
  Zero-Order Hold/1 -> q rounder16/1(in)
  Sum6/1 -> Unit Delay2/1
  Unit Delay2/1 -> Ad(1,3)/1(in), Ad(3,3)/1(in), Ad(2,3)/1(in), Cd(3)/1(in)
  Ad(1,2)/1(out) -> q rounder8/1(in)
  Ad(1,1)/1(out) -> q rounder7/1(in)
  Ad(2,1)/1(out) -> q rounder10/1(in)
  Ad(2,3)/1(out) -> q rounder12/1(in)
  Ad(2,2)/1(out) -> q rounder11/1(in)
  Ad(3,2)/1(out) -> q rounder14/1(in)
  Ad(3,1)/1(out) -> q rounder13/1(in)
  Ad(3,3)/1(out) -> q rounder15/1(in)
  Add2/1 -> Sum1/2
  Add3/1 -> Sum6/2
  q rounder3/1(out) -> Sum6/1
  q rounder4/1(out) -> Add4/1
  q rounder5/1(out) -> Add4/2
  q rounder6/1(out) -> Add4/3
  q rounder7/1(out) -> Add1/1
  q rounder8/1(out) -> Add1/2
  q rounder9/1(out) -> Add1/3
  q rounder10/1(out) -> Add2/1
  q rounder11/1(out) -> Add2/2
  q rounder12/1(out) -> Add2/3
  q rounder13/1(out) -> Add3/1
  q rounder14/1(out) -> Add3/2
  q rounder15/1(out) -> Add3/3
  Bd(1)/1(out) -> q rounder1/1(in)
  Cd(1)/1(out) -> q rounder4/1(in)
  Bd(2)/1(out) -> q rounder2/1(in)
  Bd(3)/1(out) -> q rounder3/1(in)
  Cd(3)/1(out) -> q rounder6/1(in)
  Cd(2)/1(out) -> q rounder5/1(in)
  Ad(1,3)/1(out) -> q rounder9/1(in)
  q rounder16/1(out) -> Bd(3)/1(in), Bd(2)/1(in), Dd/1(in), Bd(1)/1(in)
  q rounder17/1(out) -> Sum5/1
  Add4/1 -> Sum5/2
  Add1/1 -> Sum/2
  q rounder1/1(out) -> Sum/1
  filter in/1 -> Zero-Order Hold/1
  q rounder2/1(out) -> Sum1/1

== system general_charger_2_precharge/control_stage/AC//DC Control ==
  vac : Inport
  vdc : Inport  Port=2
  iac : Inport  Port=3
  Constant : Constant  Value=acdc_control
  Constant1 : Constant  Value=0
  Constant2 : Constant  Value=0
  DQ Controller : Subsystem
  Full Birdge IGBT drivers : Subsystem
  Multiport Switch : MultiPortSwitch
  Mux : Mux  Inputs=3
  Mux1 : Mux  Inputs=3
  PI Controller : Subsystem  mask{vdc_ref=dc_volt, vdc_ki=pi_vdc_ki, vdc_kp=pi_vdc_kp, iac_ki=pi_iac_ki, iac_kp=pi_iac_kp, vac_scale=ac_volt, Ts=switch_Ts, turn_on=reactive_power_on}
      mask prompts: vdc_ref "Vdc Reference Voltage"; vdc_ki "Vdc Integral Gain"; vdc_kp "Vdc Proportional Gain"; iac_ki "Iac Integral Gain"; iac_kp "Iac Proportional Gain"; vac_scale "ACV Peak Value"; Ts "Sample Time"; turn_on "Reactive Power Turn ON"
  PR Controller : Subsystem  mask{vdc_ref=dc_volt, ac_peak=ac_volt, vdc_ki=pr_vdc_ki, vdc_kp=pr_vdc_kp, pr_ki=pr_pr_ki, pr_kp=pr_pr_kp, iac_kp=pr_iac_kp, Ts=switch_Ts, f=60, turn_on=reactive_power_on}
      mask prompts: vdc_ref "reference voltage"; ac_peak "peak ac voltage"; vdc_ki "vdc integral gain"; vdc_kp "vdc proportional gain"; pr_ki "pr integral gain"; pr_kp "pr proportional gain"; iac_kp "iac proportional gain"; Ts "Sample Time"; f "Frequency"; turn_on "reactive power turn on"
  Scope : Scope
      settings: SaveName=ScopeData14
  Step : Step  Time=0  SampleTime=0
  Switch : Switch  Threshold=0.5
  wires:
  Constant/1 -> Multiport Switch/1
  vac/1 -> Mux/1
  vdc/1 -> Mux/2
  iac/1 -> Mux/3
  Multiport Switch/1 -> Scope/1, Full Birdge IGBT drivers/1(v_cont)
  DQ Controller/1(v_cont) -> Multiport Switch/3
  PR Controller/1(v_cont) -> Multiport Switch/4
  PI Controller/1(Vmod) -> Multiport Switch/2
  Constant1/1 -> Mux1/3, Mux1/1, Mux1/2
  Mux/1 -> Switch/1
  Mux1/1 -> Switch/3
  Switch/1 -> DQ Controller/1(inputs), PI Controller/1(inputs), PR Controller/1(inputs)
  Step/1 -> Switch/2

== system general_charger_2_precharge/control_stage/DC//DC Control ==
  Ibatt : Inport
  Vbatt : Inport  Port=2
  Add : Sum  Inputs=-+
  Add1 : Sum  Inputs=+-
  Add2 : Sum  Inputs=+-
  Add3 : Sum  Inputs=+-
  Constant1 : Constant  Value=cv_ref
  Constant2 : Constant  Value=mode
  Constant3 : Constant  Value=cc_ref
  Constant5 : Constant  Value=P
  Multiport Switch : MultiPortSwitch
  PI1 : Subsystem  mask{ki=cc_ki, kp=cc_kp, Ts_pi=Ts, int_sat_up=inf, int_sat_low=-inf, pi_sat_up=inf, pi_sat_low=-inf, pi_on=pturn_on}
      mask prompts: ki "Integral Gain"; kp "Proportional Gain"; Ts_pi "Sample Time"; int_sat_up "Integral Saturation Upper"; int_sat_low "Integral Saturation Lower"; pi_sat_up "PI Controller Saturation Upper"; pi_sat_low "PI Controller Saturation Lower"; pi_on "PI Controller Turn on Time, s"
      mask Display: disp('PI')
  PI2 : Subsystem  mask{ki=vc_ki, kp=vc_kp, Ts_pi=Ts, int_sat_up=inf, int_sat_low=-inf, pi_sat_up=inf, pi_sat_low=-inf, pi_on=turn_on}
      mask prompts: ki "Integral Gain"; kp "Proportional Gain"; Ts_pi "Sample Time"; int_sat_up "Integral Saturation Upper"; int_sat_low "Integral Saturation Lower"; pi_sat_up "PI Controller Saturation Upper"; pi_sat_low "PI Controller Saturation Lower"; pi_on "PI Controller Turn on Time, s"
      mask Display: disp('PI')
  PI3 : Subsystem  mask{ki=cc_ki, kp=cc_kp, Ts_pi=Ts, int_sat_up=inf, int_sat_low=-inf, pi_sat_up=inf, pi_sat_low=-inf, pi_on=turn_on}
      mask prompts: ki "Integral Gain"; kp "Proportional Gain"; Ts_pi "Sample Time"; int_sat_up "Integral Saturation Upper"; int_sat_low "Integral Saturation Lower"; pi_sat_up "PI Controller Saturation Upper"; pi_sat_low "PI Controller Saturation Lower"; pi_on "PI Controller Turn on Time, s"
      mask Display: disp('PI')
  PI4 : Subsystem  mask{ki=P_ki, kp=P_kp, Ts_pi=Ts, int_sat_up=inf, int_sat_low=-inf, pi_sat_up=inf, pi_sat_low=-inf, pi_on=pturn_on}
      mask prompts: ki "Integral Gain"; kp "Proportional Gain"; Ts_pi "Sample Time"; int_sat_up "Integral Saturation Upper"; int_sat_low "Integral Saturation Lower"; pi_sat_up "PI Controller Saturation Upper"; pi_sat_low "PI Controller Saturation Lower"; pi_on "PI Controller Turn on Time, s"
      mask Display: disp('PI')
  Saturation2 : Saturate  UpperLimit=1  LowerLimit=-1
  half bridge control : Subsystem
  wires:
  Vbatt/1 -> Add1/2
  Add/1 -> PI1/1(in)
  Multiport Switch/1 -> Saturation2/1
  [power] -> Add2/2
  Add1/1 -> PI2/1(in)
  Add2/1 -> PI4/1(in)
  Saturation2/1 -> half bridge control/1(v_cont)
  PI2/1(out) -> Multiport Switch/2
  Constant2/1 -> Multiport Switch/1
  Constant1/1 -> Add1/1
  PI1/1(out) -> Multiport Switch/4
  Add3/1 -> PI3/1(in)
  Constant3/1 -> Add3/1
  PI3/1(out) -> Multiport Switch/3
  Ibatt/1 -> Add3/2, Add/1
  PI4/1(out) -> Add/2
  Constant5/1 -> Add2/1

== system general_charger_2_precharge/Measurements/Power and angle calculations/AB-DQ Transform ==
  Va : Inport
  Ia : Inport  Port=2
  phi : Inport  Port=3
  Iab_dq : Subsystem  mask{abdq_f=60, abdq_Ts=switch_Ts}
      mask prompts: abdq_f "frequency"; abdq_Ts "Sample Time"
      mask init:
      | SpC=1/abdq_f/4/abdq_Ts;
      | RSpC=ceil(SpC);
  Vab_dq : Subsystem  mask{pll_f=60, pll_Ts=switch_Ts, pll_ki=50, pll_kp=5}
      mask prompts: pll_f "frequency"; pll_Ts "Sample Time"; pll_ki "PI Integral Gain"; pll_kp "PI Proportional Gain"
  Vd : Outport
  Vq : Outport  Port=2
  Id : Outport  Port=3
  Iq : Outport  Port=4
  theta : Outport  Port=5
  wires:
  phi/1 -> Iab_dq/3(phi)
  Va/1 -> Vab_dq/1(signal_in)
  Ia/1 -> Iab_dq/1(A)
  Vab_dq/2(D) -> Vd/1
  Vab_dq/3(Q) -> Vq/1
  Vab_dq/1(angle_out) -> Iab_dq/2(wt), theta/1
  Iab_dq/1(D) -> Id/1
  Iab_dq/2(Q) -> Iq/1

== system general_charger_2_precharge/Measurements/Power and angle calculations/DC Pass Filter (1st Order) ==
  u[k] : Inport
  A : Gain  Gain=dcAd
  B : Gain  Gain=dcBd
  C : Gain  Gain=dcCd
  D : Gain  Gain=dcDd
  Delay : Delay  DelayLength=1  InitialCondition=0  SampleTime=5e-5
  Sum : Sum  Inputs=|++
  Sum1 : Sum  Inputs=|++
  y[k] : Outport
  wires:
  B/1 -> Sum/1
  u[k]/1 -> D/1, B/1
  Sum1/1 -> y[k]/1
  Delay/1 -> A/1, C/1
  Sum/1 -> Delay/1
  D/1 -> Sum1/1
  A/1 -> Sum/2
  C/1 -> Sum1/2

== system general_charger_2_precharge/Measurements/Power and angle calculations/DC Pass Filter (1st Order)1 ==
  u[k] : Inport
  A : Gain  Gain=dcAd
  B : Gain  Gain=dcBd
  C : Gain  Gain=dcCd
  D : Gain  Gain=dcDd
  Delay : Delay  DelayLength=1  InitialCondition=0  SampleTime=5e-5
  Sum : Sum  Inputs=|++
  Sum1 : Sum  Inputs=|++
  y[k] : Outport
  wires:
  B/1 -> Sum/1
  u[k]/1 -> D/1, B/1
  Sum1/1 -> y[k]/1
  Delay/1 -> A/1, C/1
  Sum/1 -> Delay/1
  D/1 -> Sum1/1
  A/1 -> Sum/2
  C/1 -> Sum1/2

== system general_charger_2_precharge/Measurements/Power and angle calculations/RMS1 ==
  ac in : Inport
  Constant : Constant  Value=K1
  Constant1 : Constant  Value=f  SampleTime=-1
  Constant2 : Constant  Value=K2
  Delay : Delay  DelayLength=ceil(SpC)  SampleTime=rms_Ts
  Gain : Gain  Gain=K1  SaturateOnIntegerOverflow=on  OutDataTypeStr=Inherit: Same as input  ParamDataTypeStr=Inherit: Same as input
  Gain1 : Gain  Gain=K2  SaturateOnIntegerOverflow=on  OutDataTypeStr=Inherit: Same as input  ParamDataTypeStr=Inherit: Same as input
  PI3 : Subsystem  mask{ki=1, kp=0, Ts_pi=rms_Ts, int_sat_up=inf, int_sat_low=-inf, pi_sat_up=inf, pi_sat_low=-inf}
      mask prompts: ki "Integral Gain"; kp "Proportional Gain"; Ts_pi "Sample Time"; int_sat_up "Integral Saturation Upper"; int_sat_low "Integral Saturation Lower"; pi_sat_up "PI Controller Saturation Upper"; pi_sat_low "PI Controller Saturation Lower"
      mask Display: disp('PI')
  Product3 : Product  SaturateOnIntegerOverflow=on  InputSameDT=on  OutDataTypeStr=Inherit: Same as first input
  Product4 : Product  SaturateOnIntegerOverflow=on  InputSameDT=on  OutDataTypeStr=Inherit: Same as first input
  Pulse Generator : DiscretePulseGenerator  Period=rms_Ts/sys_Ts  SampleTime=sys_Ts
  Sample and Hold : powerlib_meascontrol/Additional Components/Sample and Hold  ic=0  Ts=sys_Ts
  Saturation : Saturate  UpperLimit=inf  LowerLimit=0
  Scope : Scope  NumInputPorts=2
      settings: YMin=-5~-5  YMax=5~5  SaveName=ScopeData2
  Sqrt : Sqrt  SaturateOnIntegerOverflow=on
  Sum1 : Sum  Inputs=+-  SaturateOnIntegerOverflow=on  InputSameDT=on  OutDataTypeStr=Inherit: Same as first input
  Sum2 : Sum  Inputs=-+  SaturateOnIntegerOverflow=on  InputSameDT=on  OutDataTypeStr=Inherit: Same as first input
  Sum3 : Sum  SaturateOnIntegerOverflow=on  InputSameDT=on  OutDataTypeStr=Inherit: Same as first input
  Unit Delay : UnitDelay  SampleTime=rms_Ts
  rms out : Outport
  wires:
  Sum2/1 -> Product4/1
  Constant1/1 -> Product4/2
  Delay/1 -> Sum2/1
  Product3/1 -> Unit Delay/1, Gain1/1, PI3/1(in)
  PI3/1(out) -> Sum2/2, Delay/1
  Sqrt/1 -> rms out/1
  Gain1/1 -> Sum1/1
  Unit Delay/1 -> Gain/1
  Gain/1 -> Sum1/2
  Product4/1 -> Sum3/1
  Sum3/1 -> Saturation/1
  Sum1/1 -> Sum3/2  "Correction"
  Saturation/1 -> Sqrt/1
  Pulse Generator/1 -> Sample and Hold/2
  Sample and Hold/1 -> Product3/1, Product3/2
  ac in/1 -> Sample and Hold/1
  Constant2/1 -> Scope/2
  Constant/1 -> Scope/1

== system general_charger_2_precharge/Measurements/Power and angle calculations/RMS4 ==
  ac in : Inport
  Constant : Constant  Value=K1
  Constant1 : Constant  Value=f  SampleTime=-1
  Constant2 : Constant  Value=K2
  Delay : Delay  DelayLength=ceil(SpC)  SampleTime=rms_Ts
  Gain : Gain  Gain=K1  SaturateOnIntegerOverflow=on  OutDataTypeStr=Inherit: Same as input  ParamDataTypeStr=Inherit: Same as input
  Gain1 : Gain  Gain=K2  SaturateOnIntegerOverflow=on  OutDataTypeStr=Inherit: Same as input  ParamDataTypeStr=Inherit: Same as input
  PI3 : Subsystem  mask{ki=1, kp=0, Ts_pi=rms_Ts, int_sat_up=inf, int_sat_low=-inf, pi_sat_up=inf, pi_sat_low=-inf}
      mask prompts: ki "Integral Gain"; kp "Proportional Gain"; Ts_pi "Sample Time"; int_sat_up "Integral Saturation Upper"; int_sat_low "Integral Saturation Lower"; pi_sat_up "PI Controller Saturation Upper"; pi_sat_low "PI Controller Saturation Lower"
      mask Display: disp('PI')
  Product3 : Product  SaturateOnIntegerOverflow=on  InputSameDT=on  OutDataTypeStr=Inherit: Same as first input
  Product4 : Product  SaturateOnIntegerOverflow=on  InputSameDT=on  OutDataTypeStr=Inherit: Same as first input
  Pulse Generator : DiscretePulseGenerator  Period=rms_Ts/sys_Ts  SampleTime=sys_Ts
  Sample and Hold : powerlib_meascontrol/Additional Components/Sample and Hold  ic=0  Ts=sys_Ts
  Saturation : Saturate  UpperLimit=inf  LowerLimit=0
  Scope : Scope  NumInputPorts=2
      settings: YMin=-5~-5  YMax=5~5  SaveName=ScopeData2
  Sqrt : Sqrt  SaturateOnIntegerOverflow=on
  Sum1 : Sum  Inputs=+-  SaturateOnIntegerOverflow=on  InputSameDT=on  OutDataTypeStr=Inherit: Same as first input
  Sum2 : Sum  Inputs=-+  SaturateOnIntegerOverflow=on  InputSameDT=on  OutDataTypeStr=Inherit: Same as first input
  Sum3 : Sum  SaturateOnIntegerOverflow=on  InputSameDT=on  OutDataTypeStr=Inherit: Same as first input
  Unit Delay : UnitDelay  SampleTime=rms_Ts
  rms out : Outport
  wires:
  Sum2/1 -> Product4/1
  Constant1/1 -> Product4/2
  Delay/1 -> Sum2/1
  Product3/1 -> Unit Delay/1, Gain1/1, PI3/1(in)
  PI3/1(out) -> Sum2/2, Delay/1
  Sqrt/1 -> rms out/1
  Gain1/1 -> Sum1/1
  Unit Delay/1 -> Gain/1
  Gain/1 -> Sum1/2
  Product4/1 -> Sum3/1
  Sum3/1 -> Saturation/1
  Sum1/1 -> Sum3/2  "Correction"
  Saturation/1 -> Sqrt/1
  Pulse Generator/1 -> Sample and Hold/2
  Sample and Hold/1 -> Product3/1, Product3/2
  ac in/1 -> Sample and Hold/1
  Constant2/1 -> Scope/2
  Constant/1 -> Scope/1
